simulink library "AEMS_Standard_Library"  (R2016b)
settings: Solver=ode45  StartTime=0.0  StopTime=10.0  RelTol=1e-3
undefined symbols (not defined in the file or in its folder): BkPY, carto, Cbx_extegr, Cbx_lpegrsys, Cbx_portegr, Cnx_bnk_nr_conf, Cnx_cyl_nr_conf, ConfigManagement, configuration_management, Cxx_dcm_io_tmr_end_xxxx, Cxx_dcm_rt_tmr_end, Cxx_DID_xxxx_IO_max, Cxx_DID_xxxx_IO_min, Cxx_egrhsofs, Cxx_vmaniegi, DEM_DEBOUNCE_FREEZE, DEM_DTR_CTL_INVISIBLE, DEM_DTR_CTL_NORMAL, Dem_DtrId2_XXX, Dem_DtrId3_XXX, Dem_DtrId4_XXX, Dem_DtrId5_XXX, Dem_DtrId6_XXX, Dem_DtrId7_XXX, Dem_DtrId8_XXX, Dem_DtrId9_XXX, Dem_DtrId_XXX, Dem_EnableConditionId2_XXX, Dem_EnableConditionId3_XXX, Dem_EnableConditionId4_XXX, Dem_EnableConditionId5_XXX, Dem_EnableConditionId6_XXX, Dem_EnableConditionId7_XXX, Dem_EnableConditionId8_XXX, Dem_EnableConditionId_XXX, Dem_EventId, Dem_EventId2_XXX, Dem_EventId3_XXX, Dem_EventId4_XXX, Dem_EventId5_XXX, Dem_EventId6_XXX, Dem_EventId7_XXX, Dem_EventId8_XXX, Dem_EventId9_XXX, Dem_EventId_Device_Faulttype, Dem_EventId_XXX, DEM_IUMPR_GENERAL_DENOMINATOR, DEM_OPCYC_IGNITION, Dem_RatioId2_XXX, Dem_RatioId3_XXX, Dem_RatioId4_XXX, Dem_RatioId5_XXX, Dem_RatioId6_XXX, Dem_RatioId7_XXX, Dem_RatioId8_XXX, Dem_RatioId_XXX, Dem_StorageConditionId2_XXX, Dem_StorageConditionId3_XXX, Dem_StorageConditionId4_XXX, Dem_StorageConditionId5_XXX ... (+65)
libraries: AEMS_Standard_Library x477, simulink x2
(part 39 of 39)

== stateflow chart AEMS_Standard_Library/BIT_OPERATION/AEMS_BIT_SET32/Chart ==
  (default) -> (junction 17) : {Out =uint8(Bit1)+ uint8(Bit2)* 2+uint8(Bit3)* 4+uint8(Bit4)* 8+uint8(Bit5)* 16+uint8(Bit6)* 32+uint8(Bit7)* 64+uint8(Bit8)* 128 + uint8(Bit9)* 256+ uint8(Bit10)* 512+uint8(Bit11)* 1024+uint8(Bit12)* 2048+uint8(Bit13)* 4096+uint8(Bit14)* 8192+uint8(Bit15)* 16384+uint8(Bit16)* 32768+uint8(Bit17)*65536+ uint8(Bit18)* 131072+uint8(Bit19)* 262144+uint8(Bit20)* 524288+uint8(Bit21)*1048576 +uint8(Bit22)*2097152 +uint8(Bit23)* 4194304+uint8(Bit24)*8388608 + uint8(Bit25)* 16777216+ uint8(Bit26)* 33554432+uint8(Bit27)*67108864 +uint8(Bit28)*134217728 +uint8(Bit29)*268435456 +uint8(Bit30)* 536870912+uint8(Bit31)* 1073741824+uint8(Bit32)* 2147483648;}
  data: Bit1 input; Bit2 input; Bit3 input; Bit4 input; Bit5 input; Bit6 input; Bit7 input; Bit8 input; Out output uint32; Bit9 input; Bit10 input; Bit11 input; Bit12 input; Bit13 input; Bit14 input; Bit15 input; Bit16 input; Bit17 input; Bit18 input; Bit19 input; Bit20 input; Bit21 input; Bit22 input; Bit23 input; Bit24 input; Bit25 input; Bit26 input; Bit27 input; Bit28 input; Bit29 input; Bit30 input; Bit31 input; Bit32 input
